simulink model "MMS_ESC_K_B_classic_LOG"  (R2019b)
settings: Solver=ode4  StartTime=par.sym.TStart  StopTime=par.sym.TStop  FixedStep=par.sym.max_dt  MaxStep=par.sym.max_dt  RelTol=1e-3
undefined symbols (not defined in the file): a_B, a_K, b, B_0, B_init, k, K_0, k_B, K_init, k_K, m, N_delay, par, phase, Sat, Sat_B, T_tran, w_1_B, w_1_K, w_B, w_K, W_K, w_L_B, w_L_K, w_wav
libraries: simulink x1
settings Model: Creator=Vitù  LastModifiedBy=User
settings DataIOCC: SaveFormat=Array  SaveOutput=off  SignalLogging=off  DSMLogging=off  ReturnWorkspaceOutputs=off  TimeSaveName=TIME  OutputSaveName=Yout  OutputOption=SpecifiedOutputTimes  OutputTimes=[par.sym.TStart:par.sym.Outputdt:par.sym.TStop]
settings OptimizationCC: ExpressionDepthLimit=2147483647  LifeSpan=inf
settings DebuggingCC: UnderspecifiedInitializationDetection=Classic  MergeDetectMultiDrivingBlocksExec=none  SolverPrmCheckMsg=warning  AllowSymbolicDim=off  StateNameClashWarn=warning  SFUnexpectedBacktrackingDiag=warning  SFNoUnconditionalDefaultTransitionDiag=warning  SFExecutionAtInitializationDiag=none  ArithmeticOperatorsInVariantConditions=warning
settings HardwareCC: ProdBitPerPointer=32  ProdBitPerSizeT=32  ProdBitPerPtrDiffT=32  ProdLargestAtomicFloat=None  ProdIntDivRoundTo=Undefined  ProdEndianess=Unspecified  ProdWordSize=32  ProdHWDeviceType=32-bit Generic
settings ModelReferenceCC: PropagateSignalLabelsOutOfModel=off
settings SFSimCC: SimUseLocalCustomCode=off  CustomCodeUndefinedFunction=UseInterfaceOnly
settings RTWCC: RTWUseLocalCustomCode=off
settings CodeAppCC: StateflowObjectComments=on
settings GRTTargetCC: TargetLangStandard=C89/C90 (ANSI)  GeneratePreprocessorConditionals=Disable all
settings ConfigComp: CovMetricSettings=dw  CovHtmlReporting=on  CovSaveCumulativeToWorkspaceVar=on  CovSaveSingleToWorkspaceVar=on  CovExternalEMLEnable=off  CovSFcnEnable=off
settings SimscapeCC: SimscapeNormalizeSystem=off
settings ConfigurationSet: Description=SimMechanics 2G

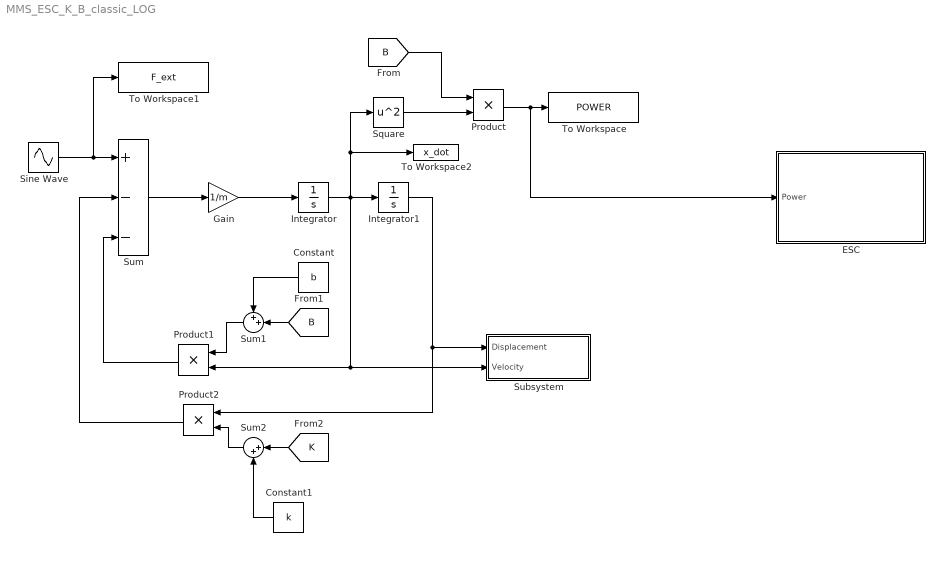
== system MMS_ESC_K_B_classic_LOG ==
  Constant : Constant  Value=b
  Constant1 : Constant  Value=k
  ESC : Subsystem
  Gain : Gain  Gain=1/m
  Integrator : Integrator
  Integrator1 : Integrator
  Product : Product
  Product1 : Product
  Product2 : Product
  Sine Wave : Sin  Amplitude=par.H  Frequency=w_wav  SampleTime=0
  Square : Math  Operator=square  SignedPower=off  SaturateOnIntegerOverflow=on
  Subsystem : Subsystem
  Sum : Sum  Inputs=+--
  Sum1 : Sum  Inputs=++|
  Sum2 : Sum  Inputs=|++
  To Workspace : ToWorkspace  VariableName=POWER  SampleTime=-1
  To Workspace1 : ToWorkspace  VariableName=F_ext  SampleTime=-1
  To Workspace2 : ToWorkspace  VariableName=x_dot  SampleTime=-1
  wires:
  Integrator1/1 -> Product2/1, Subsystem/1(Displacement)
  Product/1 -> ESC/1(Power), To Workspace/1
  Product1/1 -> Sum/3
  Gain/1 -> Integrator/1
  Square/1 -> Product/2
  Sum/1 -> Gain/1
  Integrator/1 -> Subsystem/2(Velocity), Product1/2, Square/1, To Workspace2/1, Integrator1/1
  Product2/1 -> Sum/2
  Sine Wave/1 -> To Workspace1/1, Sum/1
  [B] -> Product/1
  [B] -> Sum1/2
  Sum1/1 -> Product1/1
  Constant/1 -> Sum1/1
  [K] -> Sum2/1
  Sum2/1 -> Product2/2
  Constant1/1 -> Sum2/2

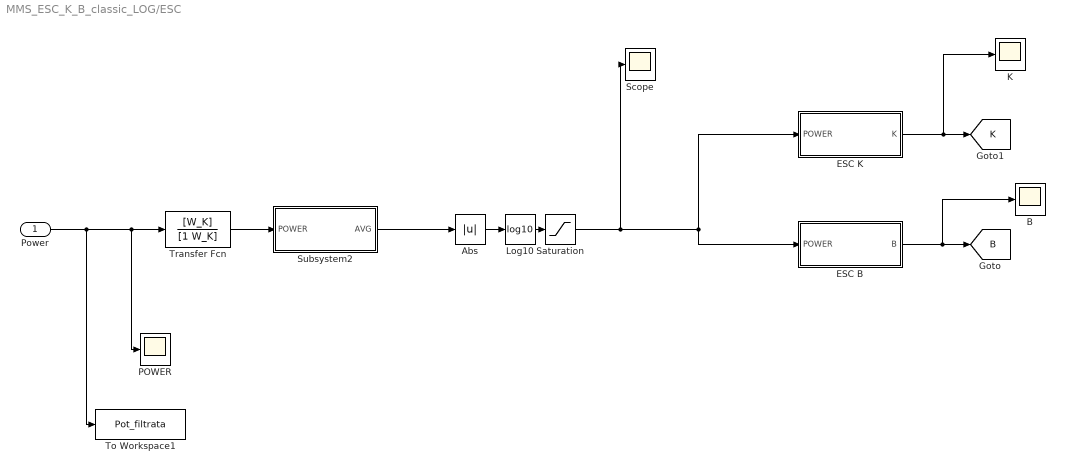
== system MMS_ESC_K_B_classic_LOG/ESC ==
  Power : Inport
  Abs : Abs
  B : Scope
  ESC B : Subsystem
  ESC K : Subsystem
  K : Scope
  Log10 : Math  Operator=log10  SignedPower=off  SaturateOnIntegerOverflow=on
  POWER : Scope
  Saturation : Saturate  UpperLimit=inf  LowerLimit=-20
  Scope : Scope
  Subsystem2 : Subsystem
  To Workspace1 : ToWorkspace  VariableName=Pot_filtrata  SampleTime=-1
  Transfer Fcn : TransferFcn  Numerator=[W_K]  Denominator=[1 W_K]
  tag scope: B=global, K=global
  wires:
  Power/1 -> Transfer Fcn/1, POWER/1, To Workspace1/1
  ESC B/1(B) -> B/1, [B]
  ESC K/1(K) -> K/1, [K]
  Saturation/1 -> Scope/1, ESC B/1(POWER), ESC K/1(POWER)
  Subsystem2/1(AVG) -> Abs/1
  Log10/1 -> Saturation/1
  Transfer Fcn/1 -> Subsystem2/1(POWER)
  Abs/1 -> Log10/1

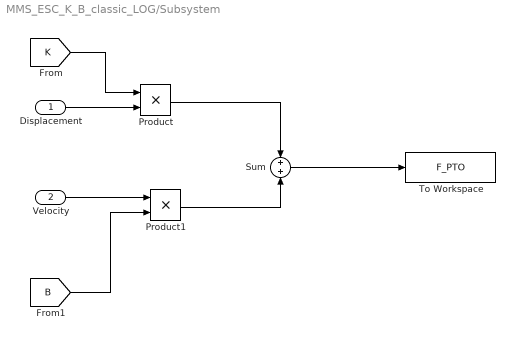
== system MMS_ESC_K_B_classic_LOG/Subsystem ==
  Displacement : Inport
  Velocity : Inport  Port=2
  Product : Product
  Product1 : Product
  Sum : Sum
  To Workspace : ToWorkspace  VariableName=F_PTO  SampleTime=-1
  wires:
  Velocity/1 -> Product1/1
  Displacement/1 -> Product/2
  [K] -> Product/1
  [B] -> Product1/2
  Product/1 -> Sum/1
  Product1/1 -> Sum/2
  Sum/1 -> To Workspace/1

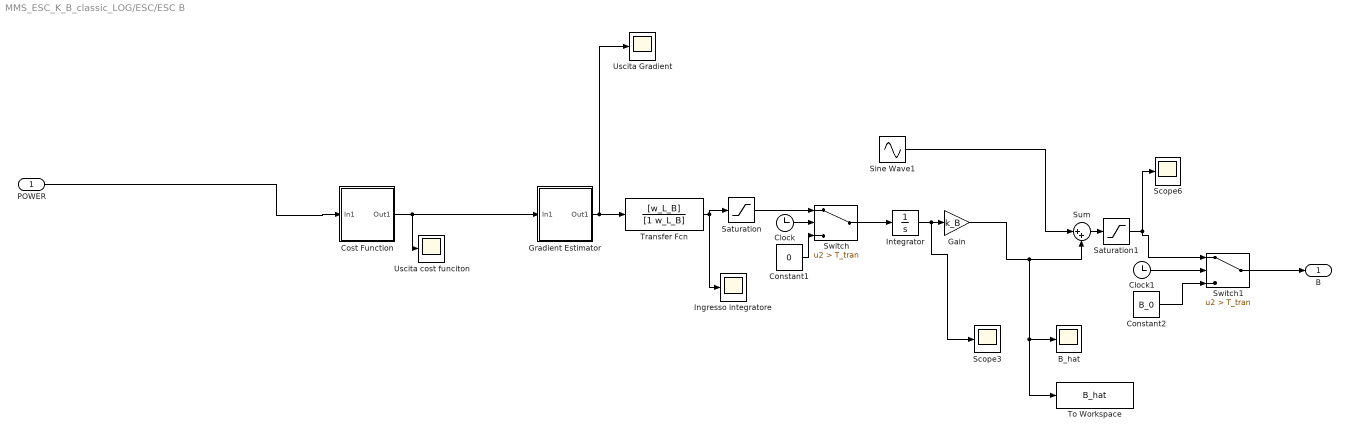
== system MMS_ESC_K_B_classic_LOG/ESC/ESC B ==
  POWER : Inport
  B_hat : Scope
  Clock : Clock
  Clock1 : Clock
  Constant1 : Constant  Value=0
  Constant2 : Constant  Value=B_0
  Cost Function : Subsystem
  Gain : Gain  Gain=k_B
  Gradient Estimator : Subsystem
  Ingresso integratore : Scope
  Integrator : Integrator  InitialCondition=B_init
  Saturation : Saturate  UpperLimit=Sat_B  LowerLimit=-Sat_B
  Saturation1 : Saturate  UpperLimit=inf  LowerLimit=-b
  Scope3 : Scope
  Scope6 : Scope
  Sine Wave1 : Sin  Amplitude=a_B  Frequency=w_B  SampleTime=0
  Sum : Sum  Inputs=|++
  Switch : Switch  Criteria=u2 > Threshold  Threshold=T_tran
  Switch1 : Switch  Criteria=u2 > Threshold  Threshold=T_tran
  To Workspace : ToWorkspace  VariableName=B_hat  SampleTime=-1
  Transfer Fcn : TransferFcn  Numerator=[w_L_B]  Denominator=[1 w_L_B]
  Uscita Gradient : Scope
  Uscita cost funciton : Scope
  B : Outport
  wires:
  Sine Wave1/1 -> Sum/1
  Gain/1 -> Sum/2, B_hat/1, To Workspace/1
  Constant2/1 -> Switch1/3
  Gradient Estimator/1(Out1) -> Transfer Fcn/1, Uscita Gradient/1
  Transfer Fcn/1 -> Saturation/1, Ingresso integratore/1
  POWER/1 -> Cost Function/1(In1)
  Cost Function/1(Out1) -> Uscita cost funciton/1, Gradient Estimator/1(In1)
  Integrator/1 -> Scope3/1, Gain/1
  Sum/1 -> Saturation1/1
  Clock1/1 -> Switch1/2
  Switch1/1 -> B/1
  Constant1/1 -> Switch/3
  Clock/1 -> Switch/2
  Switch/1 -> Integrator/1
  Saturation/1 -> Switch/1
  Saturation1/1 -> Switch1/1, Scope6/1

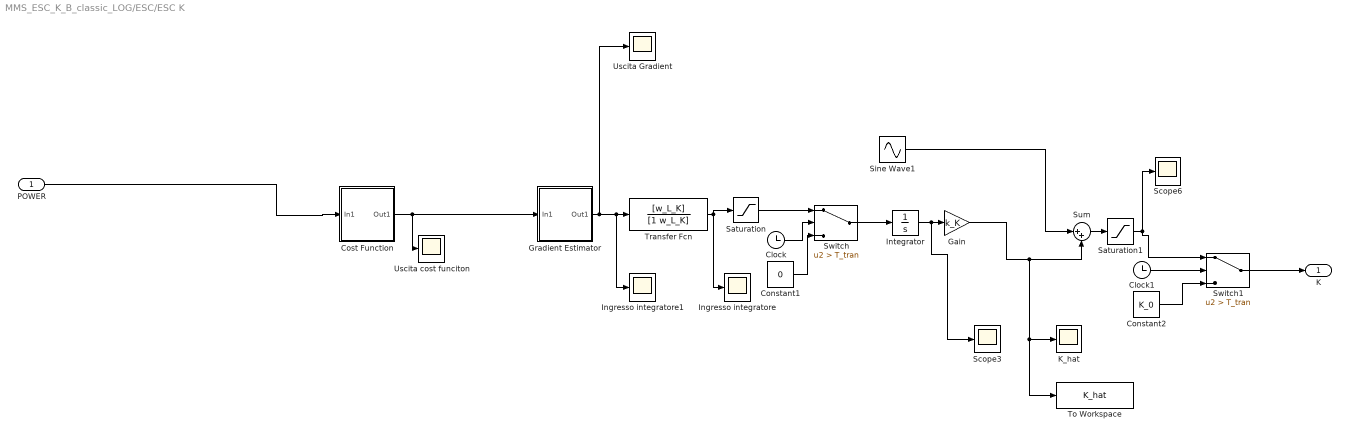
== system MMS_ESC_K_B_classic_LOG/ESC/ESC K ==
  POWER : Inport
  Clock : Clock
  Clock1 : Clock
  Constant1 : Constant  Value=0
  Constant2 : Constant  Value=K_0
  Cost Function : Subsystem
  Gain : Gain  Gain=k_K
  Gradient Estimator : Subsystem
  Ingresso integratore : Scope
  Ingresso integratore1 : Scope
  Integrator : Integrator  InitialCondition=K_init
  K_hat : Scope
  Saturation : Saturate  UpperLimit=Sat  LowerLimit=-Sat
  Saturation1 : Saturate  UpperLimit=inf  LowerLimit=-k
  Scope3 : Scope
  Scope6 : Scope
  Sine Wave1 : Sin  Amplitude=a_K  Frequency=w_K  SampleTime=0
  Sum : Sum  Inputs=|++
  Switch : Switch  Criteria=u2 > Threshold  Threshold=T_tran
  Switch1 : Switch  Criteria=u2 > Threshold  Threshold=T_tran
  To Workspace : ToWorkspace  VariableName=K_hat  SampleTime=-1
  Transfer Fcn : TransferFcn  Numerator=[w_L_K]  Denominator=[1 w_L_K]
  Uscita Gradient : Scope
  Uscita cost funciton : Scope
  K : Outport
  wires:
  Switch1/1 -> K/1
  Clock1/1 -> Switch1/2
  Sum/1 -> Saturation1/1
  Integrator/1 -> Gain/1, Scope3/1
  Cost Function/1(Out1) -> Gradient Estimator/1(In1), Uscita cost funciton/1
  POWER/1 -> Cost Function/1(In1)
  Transfer Fcn/1 -> Ingresso integratore/1, Saturation/1
  Gradient Estimator/1(Out1) -> Uscita Gradient/1, Transfer Fcn/1, Ingresso integratore1/1
  Constant2/1 -> Switch1/3
  Gain/1 -> To Workspace/1, K_hat/1, Sum/2
  Sine Wave1/1 -> Sum/1
  Clock/1 -> Switch/2
  Constant1/1 -> Switch/3
  Switch/1 -> Integrator/1
  Saturation/1 -> Switch/1
  Saturation1/1 -> Scope6/1, Switch1/1

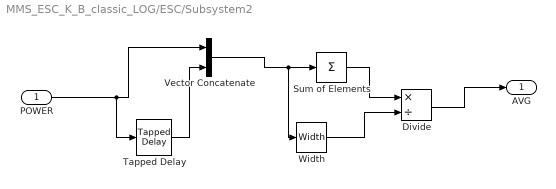
== system MMS_ESC_K_B_classic_LOG/ESC/Subsystem2 ==
  POWER : Inport
  Divide : Product  Inputs=*/
  Sum of Elements : Sum  Inputs=+
  Tapped Delay : simulink/Discrete/Tapped Delay  vinit=0  samptime=-1  NumDelays=N_delay  DelayOrder=Oldest  includeCurrent=off
  Vector Concatenate : Concatenate
  Width : Width
  AVG : Outport
  wires:
  POWER/1 -> Tapped Delay/1, Vector Concatenate/1
  Tapped Delay/1 -> Vector Concatenate/2
  Vector Concatenate/1 -> Width/1, Sum of Elements/1
  Sum of Elements/1 -> Divide/1
  Width/1 -> Divide/2
  Divide/1 -> AVG/1

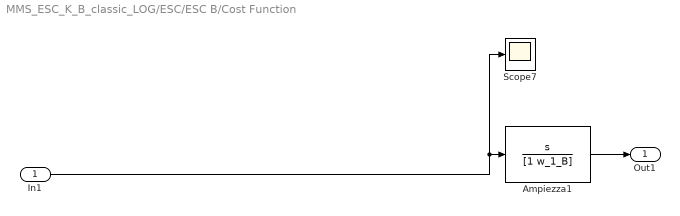
== system MMS_ESC_K_B_classic_LOG/ESC/ESC B/Cost Function ==
  In1 : Inport
  Ampiezza1 : TransferFcn  Numerator=[1 0]  Denominator=[1 w_1_B]
  Scope7 : Scope
  Out1 : Outport
  wires:
  In1/1 -> Scope7/1, Ampiezza1/1
  Ampiezza1/1 -> Out1/1

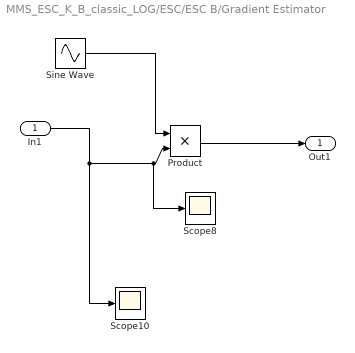
== system MMS_ESC_K_B_classic_LOG/ESC/ESC B/Gradient Estimator ==
  In1 : Inport
  Product : Product
  Scope10 : Scope
  Scope8 : Scope
  Sine Wave : Sin  Frequency=w_B  Phase=phase  SampleTime=0
  Out1 : Outport
  wires:
  In1/1 -> Scope8/1, Product/2, Scope10/1
  Sine Wave/1 -> Product/1
  Product/1 -> Out1/1

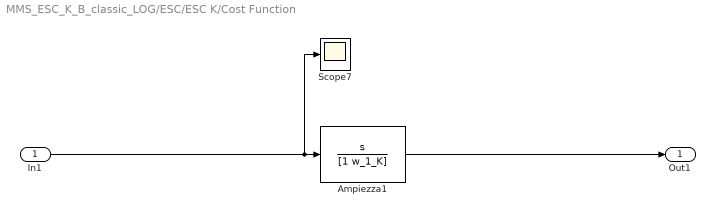
== system MMS_ESC_K_B_classic_LOG/ESC/ESC K/Cost Function ==
  In1 : Inport
  Ampiezza1 : TransferFcn  Numerator=[1 0]  Denominator=[1 w_1_K]
  Scope7 : Scope
  Out1 : Outport
  wires:
  Ampiezza1/1 -> Out1/1
  In1/1 -> Ampiezza1/1, Scope7/1

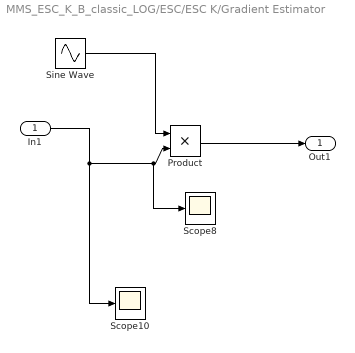
== system MMS_ESC_K_B_classic_LOG/ESC/ESC K/Gradient Estimator ==
  In1 : Inport
  Product : Product
  Scope10 : Scope
  Scope8 : Scope
  Sine Wave : Sin  Frequency=w_K  Phase=phase  SampleTime=0
  Out1 : Outport
  wires:
  Product/1 -> Out1/1
  Sine Wave/1 -> Product/1
  In1/1 -> Scope10/1, Product/2, Scope8/1
